simulink model "Test_Server"  (Simulink 7.6)
settings: Solver=ode4  SolverMode=SingleTasking  StartTime=0.0  StopTime=inf  FixedStep=0.001  MaxStep=1e-2  RelTol=1e-3
settings Model: Creator=jordan  LastModifiedBy=jordan
settings DataIOCC: LimitDataPoints=off  SaveOutput=off  SignalLogging=off  DSMLogging=off  SaveTime=off
settings OptimizationCC: OptimizeModelRefInitCode=on  LifeSpan=Inf
settings HardwareCC: ProdIntDivRoundTo=Zero  ProdEndianess=LittleEndian  ProdHWDeviceType=Generic->32-bit x86 compatible
settings RTWCC: SystemTargetFile=ert.tlc  TemplateMakefile=RTW.MSVCBuild  Description=Create Visual C/C++ Solution File for the Real-Time Workshop Embedded Coder  ProcessScript=ert_make_rtw_hook  RTWCompilerOptimization=On
settings CodeAppCC: IgnoreCustomStorageClasses=off  MaxIdLength=95
settings ERTTargetCC: MultiwordLength=2048  GenerateSampleERTMain=on  LogVarNameModifier=none  MatFileLogging=on  SupportContinuousTime=on  SupportNonInlinedSFcns=on  ERTCustomFileTemplate=example_file_process.tlc  ConvertIfToSwitch=off

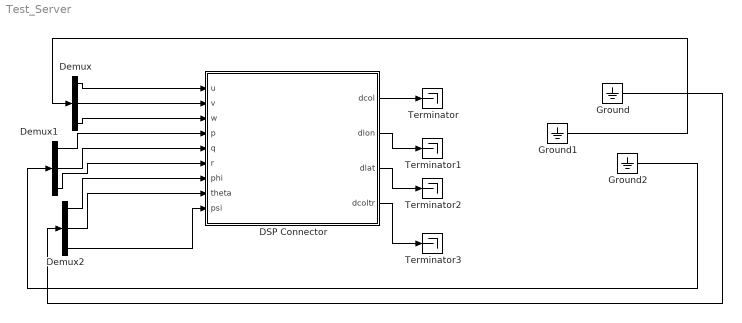
== system Test_Server ==
  DSP Connector : Subsystem
  Demux : Demux  Outputs=3
  Demux1 : Demux  Outputs=3
  Demux2 : Demux  Outputs=3
  Ground : Ground
  Ground1 : Ground
  Ground2 : Ground
  Terminator{,1..3} (4 alike) : Terminator
  wires:
  Ground1/1 -> Demux/1
  Ground2/1 -> Demux1/1
  Ground/1 -> Demux2/1
  Demux/1 -> DSP Connector/1(u)
  Demux/2 -> DSP Connector/2(v)
  Demux/3 -> DSP Connector/3(w)
  Demux1/1 -> DSP Connector/4(p)
  Demux1/2 -> DSP Connector/5(q)
  Demux1/3 -> DSP Connector/6(r)
  Demux2/1 -> DSP Connector/7(phi)
  Demux2/2 -> DSP Connector/8(theta)
  Demux2/3 -> DSP Connector/9(psi)
  DSP Connector/1(dcol) -> Terminator/1
  DSP Connector/2(dlon) -> Terminator1/1
  DSP Connector/3(dlat) -> Terminator2/1
  DSP Connector/4(dcoltr) -> Terminator3/1

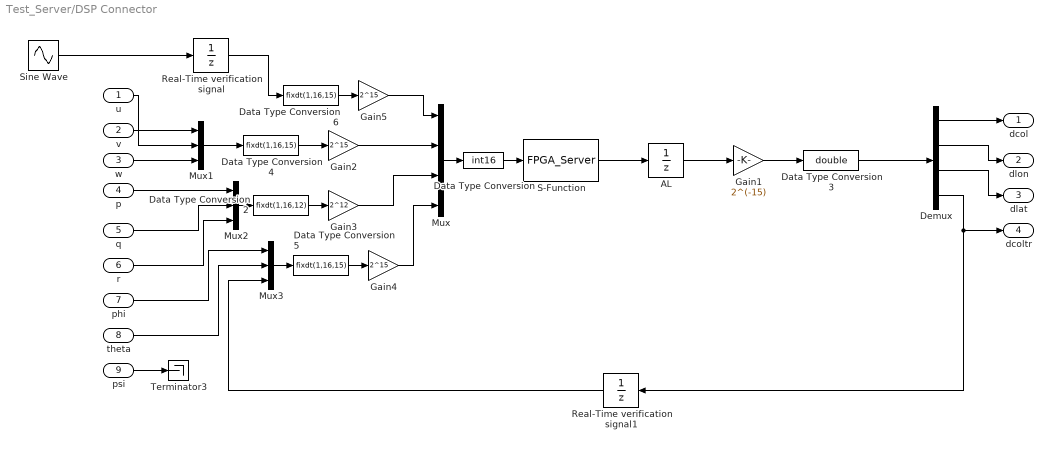
== system Test_Server/DSP Connector ==
  u : Inport
  v : Inport  Port=2
  w : Inport  Port=3
  p : Inport  Port=4
  q : Inport  Port=5
  r : Inport  Port=6
  phi : Inport  Port=7
  theta : Inport  Port=8
  psi : Inport  Port=9
  AL : UnitDelay  SampleTime=0.001
  Data Type Conversion : DataTypeConversion  OutDataTypeStr=int16  SaturateOnIntegerOverflow=on
  Data Type Conversion2 : DataTypeConversion  OutDataTypeStr=fixdt(1,16,12)  SaturateOnIntegerOverflow=on
  Data Type Conversion3 : DataTypeConversion  OutDataTypeStr=double  SaturateOnIntegerOverflow=on
  Data Type Conversion4 : DataTypeConversion  OutDataTypeStr=fixdt(1,16,15)  SaturateOnIntegerOverflow=on
  Data Type Conversion5 : DataTypeConversion  OutDataTypeStr=fixdt(1,16,15)  SaturateOnIntegerOverflow=on
  Data Type Conversion6 : DataTypeConversion  OutDataTypeStr=fixdt(1,16,15)  SaturateOnIntegerOverflow=on
  Demux : Demux
  Gain1 : Gain  Gain=2^(-15)  OutDataTypeStr=fixdt(1,16,15)
  Gain2 : Gain  Gain=2^15  OutDataTypeStr=int16  SaturateOnIntegerOverflow=on
  Gain3 : Gain  Gain=2^12  OutDataTypeStr=int16  SaturateOnIntegerOverflow=on
  Gain4 : Gain  Gain=2^15  OutDataTypeStr=int16  SaturateOnIntegerOverflow=on
  Gain5 : Gain  Gain=2^15  OutDataTypeStr=int16  SaturateOnIntegerOverflow=on
  Mux : Mux
  Mux1 : Mux  Inputs=3
  Mux2 : Mux  Inputs=3
  Mux3 : Mux  Inputs=3
  Real-Time verification signal : UnitDelay  SampleTime=0.001
  Real-Time verification signal1 : UnitDelay  SampleTime=0.001
  S-Function : S-Function  FunctionName=FPGA_Server  EnableBusSupport=off
  Sine Wave : Sin  Amplitude=0.3  Frequency=2*pi  SampleTime=0
  Terminator3 : Terminator
  dcol : Outport
  dlon : Outport  Port=2
  dlat : Outport  Port=3
  dcoltr : Outport  Port=4
  wires:
  S-Function/1 -> AL/1
  Mux/1 -> Data Type Conversion/1
  Sine Wave/1 -> Real-Time verification signal/1
  Demux/1 -> dcol/1
  Real-Time verification signal/1 -> Data Type Conversion6/1
  Data Type Conversion/1 -> S-Function/1
  Gain5/1 -> Mux/1
  u/1 -> Mux1/1
  v/1 -> Mux1/2
  w/1 -> Mux1/3
  p/1 -> Mux2/1
  q/1 -> Mux2/2
  r/1 -> Mux2/3
  phi/1 -> Mux3/1
  theta/1 -> Mux3/2
  Real-Time verification signal1/1 -> Mux3/3
  psi/1 -> Terminator3/1
  Demux/2 -> dlon/1
  Demux/3 -> dlat/1
  Demux/4 -> dcoltr/1, Real-Time verification signal1/1
  Gain1/1 -> Data Type Conversion3/1
  AL/1 -> Gain1/1
  Data Type Conversion3/1 -> Demux/1
  Data Type Conversion4/1 -> Gain2/1
  Mux1/1 -> Data Type Conversion4/1
  Gain2/1 -> Mux/2
  Data Type Conversion2/1 -> Gain3/1
  Mux2/1 -> Data Type Conversion2/1
  Gain3/1 -> Mux/3
  Data Type Conversion5/1 -> Gain4/1
  Mux3/1 -> Data Type Conversion5/1
  Gain4/1 -> Mux/4
  Data Type Conversion6/1 -> Gain5/1
